simulink model "dc_motor"  (R2022b)
settings: Solver=ode15s  StartTime=0.0  StopTime=50.0  RelTol=1e-3  EnableMultiTasking=on
PreLoadFcn:
  | % Parameters
  | J = 6;     % Rotor inertia [kg*m^2]
  | L = 1e-6;  % Armature inductance [H]
  | R = 0.3;   % Armature resistance [R]
  | k = 0.5;   % EMF constant [V*s/rad]
  | K = 0.5;   % Torque constant [N*m/A]
settings Model: Creator=jrivitus  LastModifiedBy=bensweet
settings SolverCC: AlgebraicLoopSolver=TrustRegion
settings DataIOCC: SaveFormat=Array  ReturnWorkspaceOutputs=off
settings OptimizationCC: ExpressionDepthLimit=2147483647  LifeSpan=inf
settings DebuggingCC: UnconnectedInputMsg=warning  UnconnectedOutputMsg=warning  UnconnectedLineMsg=warning  PregeneratedLibrarySubsystemCodeDiagnostic=none  SFMachineParentedDataDiag=warning
settings HardwareCC: ProdBitPerPointer=32  ProdBitPerSizeT=32  ProdBitPerPtrDiffT=32  ProdLargestAtomicFloat=None  ProdIntDivRoundTo=Undefined  ProdEndianess=Unspecified  ProdWordSize=32  ProdHWDeviceType=32-bit Generic
settings ModelReferenceCC: EnableRefExpFcnMdlSchedulingChecks=on  PropagateSignalLabelsOutOfModel=off
settings SFSimCC: SimUseLocalCustomCode=off
settings RTWCC: RTWUseLocalCustomCode=off  DLArmComputeVersion=19.05
settings CodeAppCC: StateflowObjectComments=on
settings GRTTargetCC: TargetLangStandard=C89/C90 (ANSI)  CombineOutputUpdateFcns=off  GRTInterface=on
settings ConfigComp: CovMetricSettings=dw  CovSaveCumulativeToWorkspaceVar=on  CovSaveSingleToWorkspaceVar=on  CovExternalEMLEnable=off  CovSFcnEnable=off

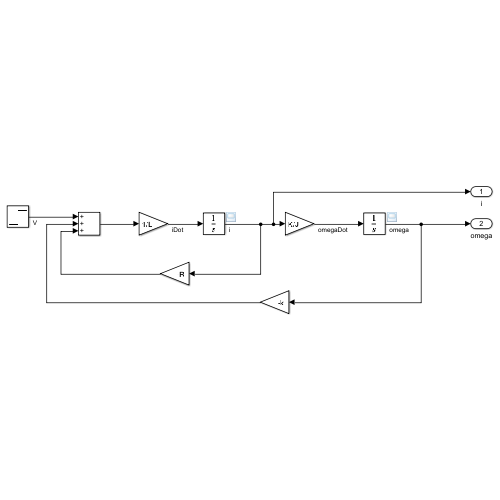
[thumbnail: Simulink's stored preview of the top-level diagram]
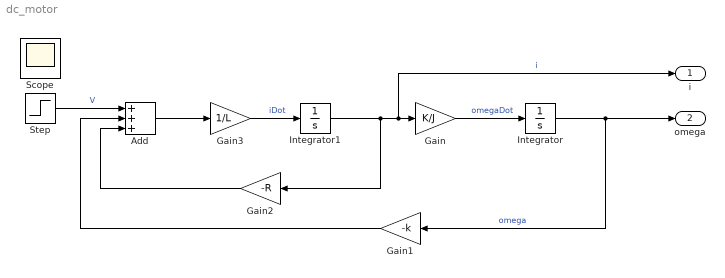
== system dc_motor ==
  Add : Sum  Inputs=+++
  Gain : Gain  Gain=K/J
  Gain1 : Gain  Gain=-k
  Gain2 : Gain  Gain=-R
  Gain3 : Gain  Gain=1/L
  Integrator : Integrator
  Integrator1 : Integrator
  Step : Step  SampleTime=0
  i : Outport  VectorParamsAs1DForOutWhenUnconnected=off
  omega : Outport  Port=2  VectorParamsAs1DForOutWhenUnconnected=off
  Scope : Scope
  wires:
  Integrator/1 -> Gain1/1, omega/1  "omega"
  Gain/1 -> Integrator/1  "omegaDot"
  Gain1/1 -> Add/2
  Step/1 -> Add/1  "V"
  Add/1 -> Gain3/1
  Integrator1/1 -> Gain2/1, i/1, Gain/1  "i"
  Gain2/1 -> Add/3
  Gain3/1 -> Integrator1/1  "iDot"
